simulink model "testor"  (R2018a)
settings: Solver=ode8  StartTime=0.0  StopTime=inf  FixedStep=1  RelTol=1e-3  EnableMultiTasking=on
InitFcn:
  | pi=22/7;
  | f = 2;
settings Model: Creator=timothy  LastModifiedBy=timothy
settings DataIOCC: LimitDataPoints=on  SaveFormat=Array
settings OptimizationCC: LifeSpan=inf
settings DebuggingCC: SFUnexpectedBacktrackingDiag=warning  SFNoUnconditionalDefaultTransitionDiag=warning  SFExecutionAtInitializationDiag=none
settings HardwareCC: ProdBitPerPointer=32  ProdBitPerSizeT=32  ProdBitPerPtrDiffT=32  ProdLargestAtomicFloat=None  ProdIntDivRoundTo=Undefined  ProdEndianess=Unspecified  ProdWordSize=32  ProdHWDeviceType=32-bit Generic
settings ModelReferenceCC: PropagateSignalLabelsOutOfModel=off
settings CodeAppCC: StateflowObjectComments=on
settings GRTTargetCC: TargetLangStandard=C89/C90 (ANSI)  GeneratePreprocessorConditionals=Disable all
settings ConfigComp: CovMetricSettings=dw  CovHtmlReporting=on  CovSaveCumulativeToWorkspaceVar=on  CovSaveSingleToWorkspaceVar=on  CovExternalEMLEnable=off

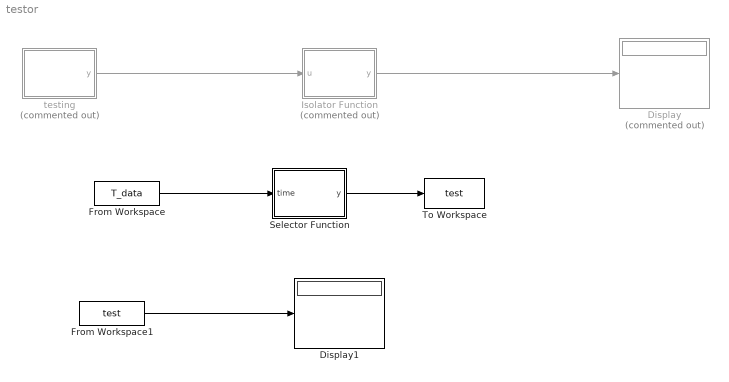
== system testor ==
  Display : Display  Commented=on
  Display1 : Display
  From Workspace : FromWorkspace  VariableName=T_data  SampleTime=0
  From Workspace1 : FromWorkspace  VariableName=test  SampleTime=0
  Isolator Function : MATLAB Function  Commented=on  TreatAsAtomicUnit=on
  Selector Function : MATLAB Function  TreatAsAtomicUnit=on
  To Workspace : ToWorkspace  VariableName=test  SaveFormat=Timeseries  SampleTime=-1
      settings: MaxDataPoints=1
  testing : MATLAB Function  Commented=on  TreatAsAtomicUnit=on
  wires:
  testing/1(y) -> Isolator Function/1(u)
  Isolator Function/1(y) -> Display/1
  Selector Function/1(y) -> To Workspace/1
  From Workspace/1 -> Selector Function/1(time)
  From Workspace1/1 -> Display1/1

== matlab function testor/Isolator Function ==
  data: u input; y output
function y = pick(u)

y = u(1);

== matlab function testor/testing ==
  data: y output
function y = testing()
 persistent t
 if isempty(t) 
     t = 0;
 end
 
 if t == 24
     t = 0;
 end
 
 if t/4 == 1
     y = [4, t/4];
 else
     y = [5, t/4];
 end
 t = t+1;

== matlab function testor/Selector Function ==
  data: time input; y output
function y = selector(time)
persistent t;
if isempty(t)
    t = 1;
end
if t == 24
    t = 1;
end

y = time(t);
t = t+1;
